simulink model "w1prob3"  (R2020a)
settings: Solver=VariableStepAuto  StartTime=0.0  StopTime=10.0  RelTol=1e-3
settings Model: Creator=Anjali123  LastModifiedBy=Anjali123

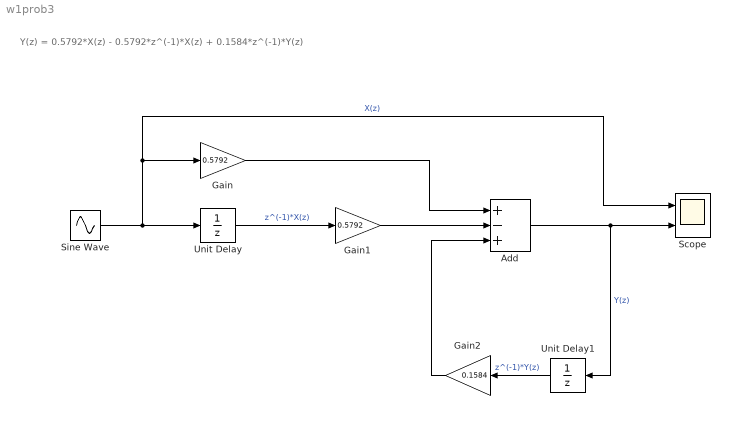
== system w1prob3 ==
  note: Y(z) = 0.5792*X(z) - 0.5792*z^(-1)*X(z) + 0.1584*z^(-1)*Y(z)
  Add : Sum  Inputs=+-+
  Gain : Gain  Gain=0.5792
  Gain1 : Gain  Gain=0.5792
  Gain2 : Gain  Gain=0.1584
  Scope : Scope  NumInputPorts=2
  Sine Wave : Sin  Frequency=100*2*pi  SampleTime=1/5000
  Unit Delay : UnitDelay  SampleTime=-1  HasFrameUpgradeWarning=on
  Unit Delay1 : UnitDelay  SampleTime=-1  HasFrameUpgradeWarning=on
  wires:
  Sine Wave/1 -> Unit Delay/1, Gain/1, Scope/1  "X(z)"
  Unit Delay/1 -> Gain1/1  "z^(-1)*X(z)"
  Add/1 -> Unit Delay1/1, Scope/2  "Y(z)"
  Gain2/1 -> Add/3
  Gain1/1 -> Add/2
  Gain/1 -> Add/1
  Unit Delay1/1 -> Gain2/1  "z^(-1)*Y(z)"
